simulink model "regressionsim"  (Simulink 7.8)
settings: Solver=ode45  StartTime=0.0  StopTime=10.0  RelTol=1e-3
libraries: dspmtrx3 x2, dspsolvers x1
settings Model: Creator=Leo  LastModifiedBy=Leo

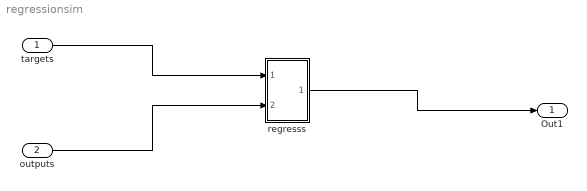
== system regressionsim ==
  targets : Inport
  outputs : Inport  Port=2
  regresss : Subsystem
  Out1 : Outport
  wires:
  targets/1 -> regresss/1(targets)
  regresss/1(Out1) -> Out1/1
  outputs/1 -> regresss/2(outputs)

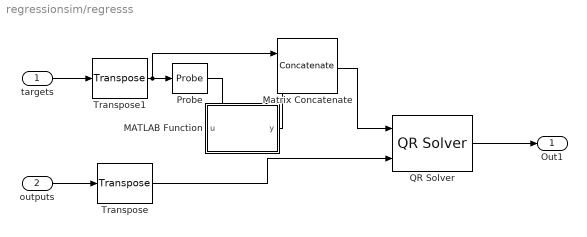
== system regressionsim/regresss ==
  targets : Inport
  outputs : Inport  Port=2
  MATLAB Function : MATLAB Function  TreatAsAtomicUnit=on
  Matrix Concatenate : Concatenate  Mode=Multidimensional array  ConcatenateDimension=2
  Probe : Probe  ProbeWidth=off  ProbeSampleTime=off  ProbeComplexSignal=off  ProbeSignalDimensions=on
  QR Solver : dspsolvers/QR Solver
  Transpose : dspmtrx3/Transpose  Hermitian=off  overflowFlag=off
  Transpose1 : dspmtrx3/Transpose  Hermitian=off  overflowFlag=off
  Out1 : Outport
  wires:
  outputs/1 -> Transpose/1
  Probe/1 -> MATLAB Function/1(u)
  targets/1 -> Transpose1/1
  Transpose1/1 -> Matrix Concatenate/1, Probe/1
  MATLAB Function/1(y) -> Matrix Concatenate/2
  Matrix Concatenate/1 -> QR Solver/1
  Transpose/1 -> QR Solver/2
  QR Solver/1 -> Out1/1

== matlab function regresss/MATLAB Function ==
  data: u input double; y output double
function y = fcn(u)
%#codegen

y = ones(u);
